simulink model "pospoli_XY"  (R2020b)
settings: Solver=ode15s  StartTime=0.0  StopTime=1.2  MaxStep=0.024  RelTol=1e-3
values from neighbouring files (symbols this model uses):
  mx = config_dc_x(parx)    [Main_Strategia_di_pilotaggio.m]    (also in Main_traiettoria.m; Main_traiettoria_ordinato.m)
  my = config_dc_y(pary)    [Main_Strategia_di_pilotaggio.m]    (also in Main_traiettoria.m; Main_traiettoria_ordinato.m)
  ppx_c = pos_poli_cc_x(mx, acx, 2)    [Main_Strategia_di_pilotaggio.m]
  ppx_m = pos_poli_cc_x(mx, acx, 1)    [Main_Strategia_di_pilotaggio.m]
  ppy_c = pos_poli_cc_y(my, acy, 2)    [Main_Strategia_di_pilotaggio.m]
  ppy_m = pos_poli_cc_y(my, acy, 1)    [Main_Strategia_di_pilotaggio.m]
undefined symbols (not defined in the file or in its folder): accelerazioni, accelerazioniy, Evaluate_Trajectory, parx, pary
settings Model: Creator=stefa  LastModifiedBy=user
settings DebuggingCC: AlgebraicLoopMsg=none  SFMachineParentedDataDiag=error

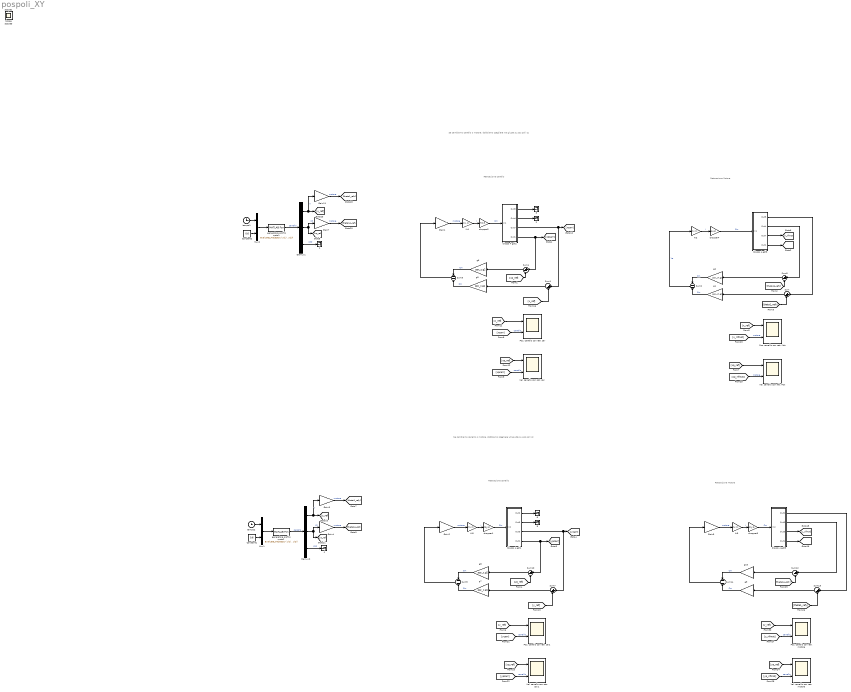
== system pospoli_XY ==
  note: Se cambiamo carrello o motore, dobbiamo scegliere w0 giusta su pos poli cc
  note: Retroazione Motore
  note: Retroazione carrello
  note: Se cambiamo carrello o motore, dobbiamo scegliere w0 giusta su pos poli cc
  note: Retroazione carrello
  note: Retroazione Motore
   {1..6} (6 alike) : Terminator
  Constant1 : Constant  Value=0.6
  Constant2 : Constant  Value=0.6
  Demux1 : Demux  Outputs=3
  Demux2 : Demux  Outputs=3
  Gain1 : Gain  Gain=1/parx.tau
  Gain11 : Gain  Gain=1/parx.tau
  Gain{2..5} (4 alike) : Gain  Gain=1/pary.tau
  Gain7 : Gain  Gain=1/parx.tau
  Kr1 : Gain  Gain=mx.Kr
  Kr2 : Gain  Gain=mx.Kr
  Kr3 : Gain  Gain=my.Kr
  Kr5 : Gain  Gain=my.Kr
  Mux1 : Mux  Inputs=2
  Mux2 : Mux  Inputs=2
  Pos. carrello con retr. Mot : Scope  NumInputPorts=2
  Pos. carrello con retr. car : Scope  NumInputPorts=2
  Pos. carrello con retr. car1 : Scope  NumInputPorts=2
  Pos. carrello con retr. motore : Scope  NumInputPorts=2
  Sum{,1,4..5,7,10,12..13} (8 alike) : Sum  Inputs=|+-
  Sum{2..3,9,14} (4 alike) : Sum  Inputs=--
  Vel. carrello con retr. Mot : Scope  NumInputPorts=2
  Vel. carrello con retr. car. : Scope  NumInputPorts=2
  Vel. carrello con retr. car.1 : Scope  NumInputPorts=2
  Vel. carrello con retr. motore : Scope  NumInputPorts=2
  blocco 4 gdl1 : Subsystem
  blocco 4 gdl2 : Subsystem
  blocco 4 gdl3 : Subsystem
  blocco 4 gdl5 : Subsystem
  chopper1 : Gain  Gain=my.K
  chopper2 : Gain  Gain=mx.K
  chopper4 : Gain  Gain=mx.K
  chopper5 : Gain  Gain=my.K
  g1 : Gain  Gain=ppx_m.g1
  g10 : Gain  Gain=ppy_m.g2
  g2 : Gain  Gain=ppx_m.g2
  g5 : Gain  Gain=ppx_c.g1
  g6 : Gain  Gain=ppx_c.g2
  g7 : Gain  Gain=ppy_c.g1
  g8 : Gain  Gain=ppy_c.g2
  g9 : Gain  Gain=ppy_m.g1
  generatore profilo moto1 : MATLABFcn  MATLABFcn=Evaluate_Trajectory( u(1) , u(2))  OutputDimensions=3
  generatore profilo moto2 : MATLABFcn  MATLABFcn=Evaluate_Trajectory( u(1) , u(2))  OutputDimensions=3
  tempo1 : Clock
  tempo2 : Clock
  Scope : Scope
  Scope1 : Scope
  Scope3 : Scope
  wires:
  [xp_ref] -> Vel. carrello con retr. Mot/1
  [x_ref] -> Pos. carrello con retr. Mot/1
  [xp_rifmot] -> Vel. carrello con retr. Mot/2  "motore"
  [x_rifmot] -> Pos. carrello con retr. Mot/2  "motore"
  Kr2/1 -> chopper4/1  "I"
  Sum2/1 -> Kr2/1  "Va"
  Sum/1 -> g1/1
  [theta1_refx] -> Sum/2
  g2/1 -> Sum2/1  "Cm"
  g1/1 -> Sum2/2  "Cm"
  [xcarr] -> Pos. carrello con retr. car/2  "carrello"
  [xpcarr] -> Vel. carrello con retr. car./2  "carrello"
  [xp_ref] -> Vel. carrello con retr. car./1
  [x_ref] -> Pos. carrello con retr. car/1
  Mux2/1 -> generatore profilo moto1/1
  Gain7/1 -> [theta1p_refx]  "motore"
  Gain11/1 -> [theta1_refx]  "motore"
  Constant2/1 -> Mux2/2
  Demux1/3 -> " 1"/1  "XPP"
  tempo1/1 -> Mux2/1
  generatore profilo moto1/1 -> Demux1/1  "carrello"
  Demux1/2 -> Gain7/1, [xp_ref]  "XP"
  Demux1/1 -> [x_ref], Gain11/1  "X"
  blocco 4 gdl3/3(Out7) -> [x_rifmot]
  chopper4/1 -> blocco 4 gdl3/1(In1)  "Cm"
  blocco 4 gdl3/4(Out1) -> [xp_rifmot]
  blocco 4 gdl3/1(Out3) -> Sum/1
  g5/1 -> Sum3/2  "Cm"
  blocco 4 gdl2/3(Out7) -> Sum1/1, [xcarr]
  [x_ref] -> Sum1/2
  chopper2/1 -> blocco 4 gdl2/1(In1)  "Cm"
  Sum1/1 -> g5/1
  Kr1/1 -> chopper2/1  "I"
  g6/1 -> Sum3/1  "Cm"
  blocco 4 gdl2/2(Out4) -> " 2"/1
  blocco 4 gdl2/1(Out3) -> " 3"/1
  Gain1/1 -> Kr1/1  "motore"
  Sum3/1 -> Gain1/1
  [xp_ref] -> Sum4/2
  blocco 4 gdl2/4(Out1) -> Sum4/1, [xpcarr]
  Sum4/1 -> g6/1
  [theta1p_refx] -> Sum5/2
  Sum5/1 -> g2/1
  blocco 4 gdl3/2(Out4) -> Sum5/1
  tempo2/1 -> Mux1/1
  generatore profilo moto2/1 -> Demux2/1  "carrello"
  Kr3/1 -> chopper1/1  "I"
  Demux2/2 -> Gain4/1, [yp_ref]  "YP"
  Constant1/1 -> Mux1/2
  Mux1/1 -> generatore profilo moto2/1
  Gain4/1 -> [theta1p_refy]  "motore"
  Sum10/1 -> g8/1
  Gain2/1 -> Kr3/1  "motore"
  [ypcarr] -> Vel. carrello con retr. car.1/2  "carrello"
  [ycarr] -> Pos. carrello con retr. car1/2  "carrello"
  blocco 4 gdl1/4(Out1) -> Sum10/1, [ypcarr]
  Sum9/1 -> Gain2/1
  g7/1 -> Sum9/2  "Cm"
  [yp_ref] -> Sum10/2
  [yp_ref] -> Vel. carrello con retr. car.1/1
  Gain3/1 -> [theta1_refy]  "motore"
  [y_ref] -> Sum7/2
  chopper1/1 -> blocco 4 gdl1/1(In2)  "Cm"
  Demux2/1 -> [y_ref], Gain3/1  "Y"
  Demux2/3 -> " 4"/1  "YPP"
  g8/1 -> Sum9/1  "Cm"
  Sum7/1 -> g7/1
  [y_ref] -> Pos. carrello con retr. car1/1
  blocco 4 gdl1/2(Out5) -> " 5"/1
  blocco 4 gdl1/1(Out2) -> " 6"/1
  blocco 4 gdl1/3(Out3) -> Sum7/1, [ycarr]
  chopper5/1 -> blocco 4 gdl5/1(In2)  "Cm"
  blocco 4 gdl5/2(Out5) -> Sum12/1
  Kr5/1 -> chopper5/1  "I"
  [yp_rifmot] -> Vel. carrello con retr. motore/2  "carrello"
  Gain5/1 -> Kr5/1  "motore"
  Sum12/1 -> g10/1
  [yp_ref] -> Vel. carrello con retr. motore/1
  [theta1p_refy] -> Sum12/2
  g9/1 -> Sum14/2  "Cm"
  Sum14/1 -> Gain5/1
  [y_ref] -> Pos. carrello con retr. motore/1
  Sum13/1 -> g9/1
  blocco 4 gdl5/1(Out2) -> Sum13/1
  g10/1 -> Sum14/1  "Cm"
  [theta1_refy] -> Sum13/2
  [y_rifmot] -> Pos. carrello con retr. motore/2  "carrello"
  blocco 4 gdl5/3(Out3) -> [y_rifmot]
  blocco 4 gdl5/4(Out1) -> [yp_rifmot]

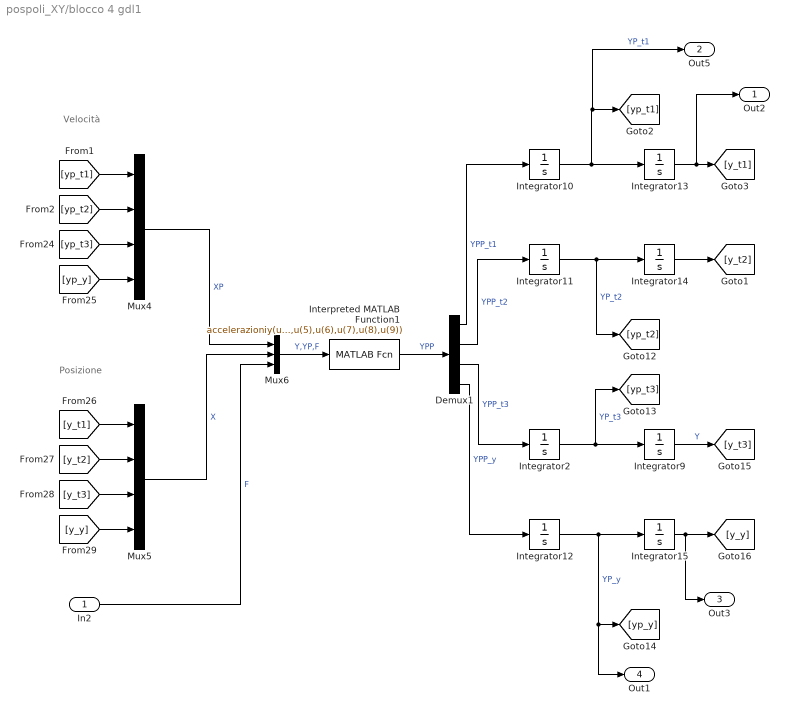
== system pospoli_XY/blocco 4 gdl1 ==
  note: Posizione
  note: Velocità
  In2 : Inport
  Demux1 : Demux
  Integrator{2,10..12} (4 alike) : Integrator
  Integrator13 : Integrator  InitialCondition=pary.Vy(1,pary.i)
  Integrator14 : Integrator  InitialCondition=pary.Vy(2,pary.i)
  Integrator15 : Integrator  InitialCondition=pary.Vy(4,pary.i)
  Integrator9 : Integrator  InitialCondition=pary.Vy(3,pary.i)
  Interpreted MATLAB Function1 : MATLABFcn  MATLABFcn=accelerazioniy(u(1),u(2),u(3),u(4),u(5),u(6),u(7),u(8),u(9))  OutputDimensions=4
  Mux4 : Mux
  Mux5 : Mux
  Mux6 : Mux  Inputs=3
  Out2 : Outport
  Out5 : Outport  Port=2
  Out3 : Outport  Port=3
  Out1 : Outport  Port=4
  wires:
  Mux4/1 -> Mux6/1  "XP"
  Integrator9/1 -> [y_t3]  "Y"
  [y_t2] -> Mux5/2
  [yp_t1] -> Mux4/1
  Integrator13/1 -> Out2/1, [y_t1]
  Demux1/4 -> Integrator12/1  "YPP_y"
  Integrator12/1 -> Out1/1, [yp_y], Integrator15/1  "YP_y"
  [yp_t3] -> Mux4/3
  Integrator2/1 -> [yp_t3], Integrator9/1  "YP_t3"
  Integrator11/1 -> [yp_t2], Integrator14/1  "YP_t2"
  Demux1/1 -> Integrator10/1  "YPP_t1"
  Integrator10/1 -> Out5/1, [yp_t1], Integrator13/1  "YP_t1"
  [y_t1] -> Mux5/1
  Mux5/1 -> Mux6/2  "X"
  [y_t3] -> Mux5/3
  Demux1/2 -> Integrator11/1  "YPP_t2"
  Interpreted MATLAB Function1/1 -> Demux1/1  "YPP"
  [yp_t2] -> Mux4/2
  [yp_y] -> Mux4/4
  Integrator14/1 -> [y_t2]
  Integrator15/1 -> Out3/1, [y_y]
  Demux1/3 -> Integrator2/1  "YPP_t3"
  Mux6/1 -> Interpreted MATLAB Function1/1  "Y,YP,F"
  [y_y] -> Mux5/4
  In2/1 -> Mux6/3  "F"

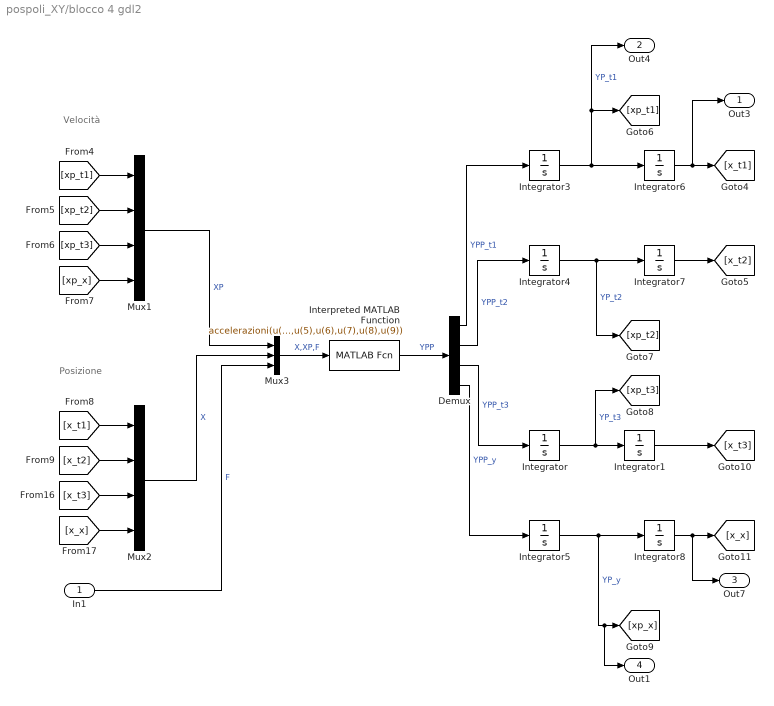
== system pospoli_XY/blocco 4 gdl2 ==
  note: Posizione
  note: Velocità
  In1 : Inport
  Demux : Demux
  Integrator{,1,3..7} (7 alike) : Integrator
  Integrator8 : Integrator  InitialCondition=0.0005
  Interpreted MATLAB Function : MATLABFcn  MATLABFcn=accelerazioni(u(1),u(2),u(3),u(4),u(5),u(6),u(7),u(8),u(9))  OutputDimensions=4
  Mux1 : Mux
  Mux2 : Mux
  Mux3 : Mux  Inputs=3
  Out3 : Outport
  Out4 : Outport  Port=2
  Out7 : Outport  Port=3
  Out1 : Outport  Port=4
  wires:
  [xp_t3] -> Mux1/3
  Interpreted MATLAB Function/1 -> Demux/1  "YPP"
  Integrator3/1 -> Out4/1, [xp_t1], Integrator6/1  "YP_t1"
  Integrator8/1 -> Out7/1, [x_x]
  Integrator7/1 -> [x_t2]
  [xp_x] -> Mux1/4
  [x_t1] -> Mux2/1
  Mux1/1 -> Mux3/1  "XP"
  [x_x] -> Mux2/4
  Demux/3 -> Integrator/1  "YPP_t3"
  Integrator/1 -> Integrator1/1, [xp_t3]  "YP_t3"
  Mux2/1 -> Mux3/2  "X"
  Integrator6/1 -> Out3/1, [x_t1]
  Integrator5/1 -> Out1/1, [xp_x], Integrator8/1  "YP_y"
  [xp_t2] -> Mux1/2
  Mux3/1 -> Interpreted MATLAB Function/1  "X,XP,F"
  [x_t3] -> Mux2/3
  In1/1 -> Mux3/3  "F"
  Demux/4 -> Integrator5/1  "YPP_y"
  Integrator4/1 -> [xp_t2], Integrator7/1  "YP_t2"
  Integrator1/1 -> [x_t3]
  [xp_t1] -> Mux1/1
  [x_t2] -> Mux2/2
  Demux/2 -> Integrator4/1  "YPP_t2"
  Demux/1 -> Integrator3/1  "YPP_t1"

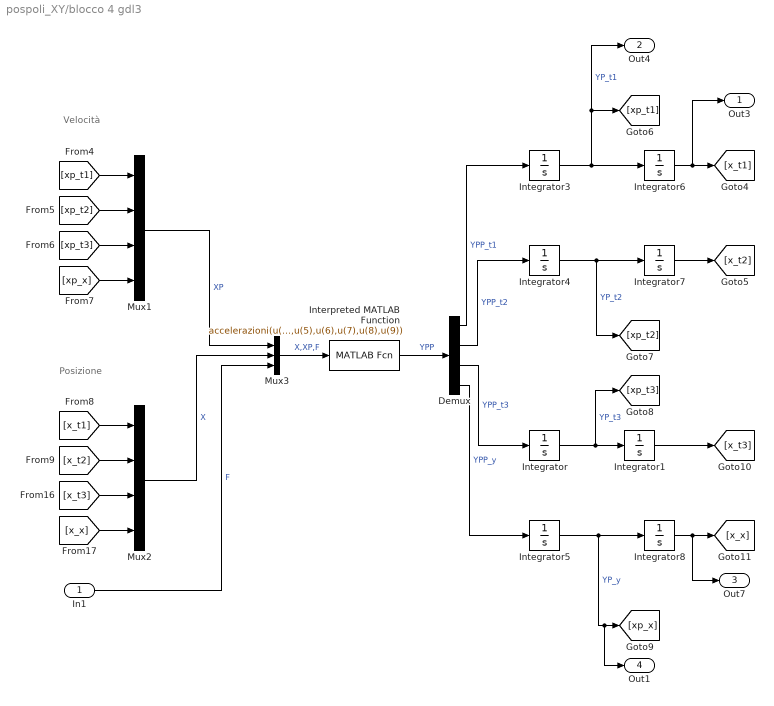
== system pospoli_XY/blocco 4 gdl3 ==
  note: Posizione
  note: Velocità
  In1 : Inport
  Demux : Demux
  Integrator{,1,3..7} (7 alike) : Integrator
  Integrator8 : Integrator  InitialCondition=0.0005
  Interpreted MATLAB Function : MATLABFcn  MATLABFcn=accelerazioni(u(1),u(2),u(3),u(4),u(5),u(6),u(7),u(8),u(9))  OutputDimensions=4
  Mux1 : Mux
  Mux2 : Mux
  Mux3 : Mux  Inputs=3
  Out3 : Outport
  Out4 : Outport  Port=2
  Out7 : Outport  Port=3
  Out1 : Outport  Port=4
  wires:
  [xp_t3] -> Mux1/3
  Interpreted MATLAB Function/1 -> Demux/1  "YPP"
  Integrator3/1 -> Out4/1, [xp_t1], Integrator6/1  "YP_t1"
  Integrator8/1 -> Out7/1, [x_x]
  Integrator7/1 -> [x_t2]
  [xp_x] -> Mux1/4
  [x_t1] -> Mux2/1
  Mux1/1 -> Mux3/1  "XP"
  [x_x] -> Mux2/4
  Demux/3 -> Integrator/1  "YPP_t3"
  Integrator/1 -> Integrator1/1, [xp_t3]  "YP_t3"
  Mux2/1 -> Mux3/2  "X"
  Integrator6/1 -> Out3/1, [x_t1]
  Integrator5/1 -> Out1/1, [xp_x], Integrator8/1  "YP_y"
  [xp_t2] -> Mux1/2
  Mux3/1 -> Interpreted MATLAB Function/1  "X,XP,F"
  [x_t3] -> Mux2/3
  In1/1 -> Mux3/3  "F"
  Demux/4 -> Integrator5/1  "YPP_y"
  Integrator4/1 -> [xp_t2], Integrator7/1  "YP_t2"
  Integrator1/1 -> [x_t3]
  [xp_t1] -> Mux1/1
  [x_t2] -> Mux2/2
  Demux/2 -> Integrator4/1  "YPP_t2"
  Demux/1 -> Integrator3/1  "YPP_t1"

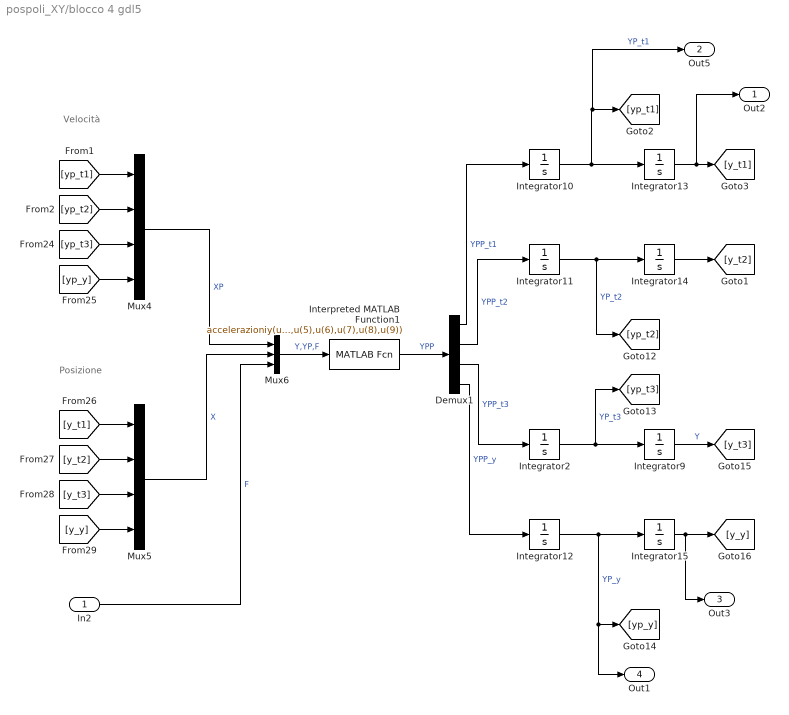
== system pospoli_XY/blocco 4 gdl5 ==
  note: Posizione
  note: Velocità
  In2 : Inport
  Demux1 : Demux
  Integrator{2,10..12} (4 alike) : Integrator
  Integrator13 : Integrator  InitialCondition=pary.Vy(1,pary.i)
  Integrator14 : Integrator  InitialCondition=pary.Vy(2,pary.i)
  Integrator15 : Integrator  InitialCondition=pary.Vy(4,pary.i)
  Integrator9 : Integrator  InitialCondition=pary.Vy(3,pary.i)
  Interpreted MATLAB Function1 : MATLABFcn  MATLABFcn=accelerazioniy(u(1),u(2),u(3),u(4),u(5),u(6),u(7),u(8),u(9))  OutputDimensions=4
  Mux4 : Mux
  Mux5 : Mux
  Mux6 : Mux  Inputs=3
  Out2 : Outport
  Out5 : Outport  Port=2
  Out3 : Outport  Port=3
  Out1 : Outport  Port=4
  wires:
  Mux4/1 -> Mux6/1  "XP"
  Integrator9/1 -> [y_t3]  "Y"
  [y_t2] -> Mux5/2
  [yp_t1] -> Mux4/1
  Integrator13/1 -> Out2/1, [y_t1]
  Demux1/4 -> Integrator12/1  "YPP_y"
  Integrator12/1 -> Out1/1, [yp_y], Integrator15/1  "YP_y"
  [yp_t3] -> Mux4/3
  Integrator2/1 -> [yp_t3], Integrator9/1  "YP_t3"
  Integrator11/1 -> [yp_t2], Integrator14/1  "YP_t2"
  Demux1/1 -> Integrator10/1  "YPP_t1"
  Integrator10/1 -> Out5/1, [yp_t1], Integrator13/1  "YP_t1"
  [y_t1] -> Mux5/1
  Mux5/1 -> Mux6/2  "X"
  [y_t3] -> Mux5/3
  Demux1/2 -> Integrator11/1  "YPP_t2"
  Interpreted MATLAB Function1/1 -> Demux1/1  "YPP"
  [yp_t2] -> Mux4/2
  [yp_y] -> Mux4/4
  Integrator14/1 -> [y_t2]
  Integrator15/1 -> Out3/1, [y_y]
  Demux1/3 -> Integrator2/1  "YPP_t3"
  Mux6/1 -> Interpreted MATLAB Function1/1  "Y,YP,F"
  [y_y] -> Mux5/4
  In2/1 -> Mux6/3  "F"
